simulink model "TST_OilPLmp_DD"  (R2016b)
settings: Solver=FixedStepDiscrete  StartTime=0.0  StopTime=simTime  FixedStep=sampleTime  RelTol=1e-3
values from neighbouring files (symbols this model uses):
  testCase = 1    [initTST_OilPLmp_DD_001.m]    (also in initTST_OilPLmp_DD_002.m = 2)
libraries: simulink x5, UnitTest_Lib x2
settings Model: Creator=xinchangran  LastModifiedBy=xinchangran
settings DebuggingCC: SignalRangeChecking=error

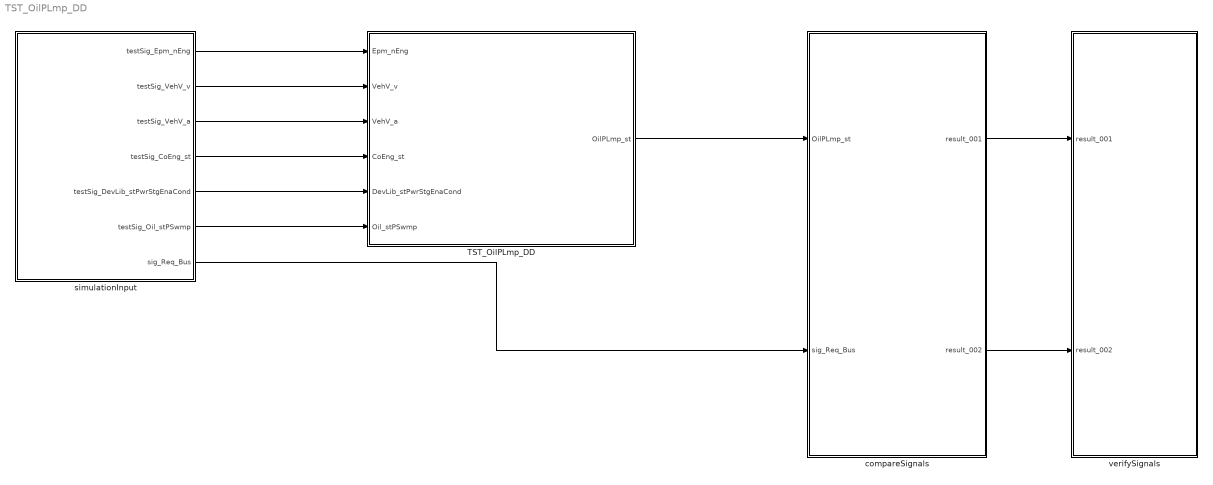
== system TST_OilPLmp_DD ==
  TST_OilPLmp_DD : Subsystem
  compareSignals : Subsystem
  simulationInput : Subsystem
  verifySignals : Subsystem
  wires:
  simulationInput/1(testSig_Epm_nEng) -> TST_OilPLmp_DD/1(Epm_nEng)
  simulationInput/2(testSig_VehV_v) -> TST_OilPLmp_DD/2(VehV_v)
  simulationInput/3(testSig_VehV_a) -> TST_OilPLmp_DD/3(VehV_a)
  simulationInput/4(testSig_CoEng_st) -> TST_OilPLmp_DD/4(CoEng_st)
  simulationInput/5(testSig_DevLib_stPwrStgEnaCond) -> TST_OilPLmp_DD/5(DevLib_stPwrStgEnaCond)
  simulationInput/6(testSig_Oil_stPSwmp) -> TST_OilPLmp_DD/6(Oil_stPSwmp)
  TST_OilPLmp_DD/1(OilPLmp_st) -> compareSignals/1(OilPLmp_st)
  simulationInput/7(sig_Req_Bus) -> compareSignals/2(sig_Req_Bus)
  compareSignals/1(result_001) -> verifySignals/1(result_001)
  compareSignals/2(result_002) -> verifySignals/2(result_002)

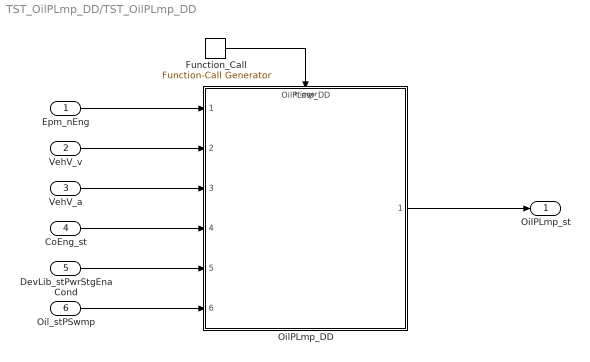
== system TST_OilPLmp_DD/TST_OilPLmp_DD ==
  Epm_nEng : Inport
  VehV_v : Inport  Port=2
  VehV_a : Inport  Port=3
  CoEng_st : Inport  Port=4
  DevLib_stPwrStgEnaCond : Inport  Port=5
  Oil_stPSwmp : Inport  Port=6
  Function_Call : simulink/Ports & Subsystems/Function-Call Generator  sample_time=sampleTime  numberOfIterations=1
  OilPLmp_DD : ModelReference  ModelNameDialog=OilPLmp_DD  SimulationMode=Normal  ModelReferenceVersion=1.211  TriggerPortName=function  TriggerPortTriggerType=function-call  TriggerPortStatesWhenEnabling=held
  OilPLmp_st : Outport
  wires:
  Function_Call/1 -> OilPLmp_DD/Trigger
  Epm_nEng/1 -> OilPLmp_DD/1
  VehV_v/1 -> OilPLmp_DD/2
  VehV_a/1 -> OilPLmp_DD/3
  CoEng_st/1 -> OilPLmp_DD/4
  DevLib_stPwrStgEnaCond/1 -> OilPLmp_DD/5
  Oil_stPSwmp/1 -> OilPLmp_DD/6
  OilPLmp_DD/1 -> OilPLmp_st/1

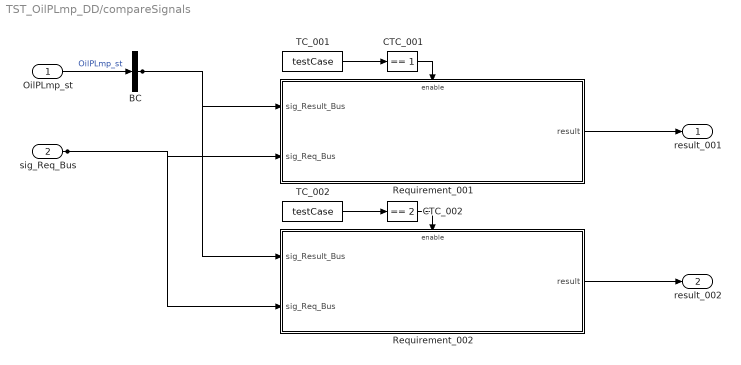
== system TST_OilPLmp_DD/compareSignals ==
  OilPLmp_st : Inport
  sig_Req_Bus : Inport  Port=2
  BC : BusCreator  Inputs=1
  CTC_001 : simulink/Logic and Bit Operations/Compare To Constant  relop===  const=1  OutDataTypeStr=boolean
  CTC_002 : simulink/Logic and Bit Operations/Compare To Constant  relop===  const=2  OutDataTypeStr=boolean
  Requirement_001 : Subsystem
  Requirement_002 : Subsystem
  TC_001 : Constant  Value=testCase
  TC_002 : Constant  Value=testCase
  result_001 : Outport
  result_002 : Outport  Port=2
  wires:
  OilPLmp_st/1 -> BC/1  "OilPLmp_st"
  TC_001/1 -> CTC_001/1
  CTC_001/1 -> Requirement_001/Enable
  sig_Req_Bus/1 -> Requirement_001/2(sig_Req_Bus), Requirement_002/2(sig_Req_Bus)
  BC/1 -> Requirement_001/1(sig_Result_Bus), Requirement_002/1(sig_Result_Bus)
  Requirement_001/1(result) -> result_001/1
  TC_002/1 -> CTC_002/1
  CTC_002/1 -> Requirement_002/Enable
  Requirement_002/1(result) -> result_002/1

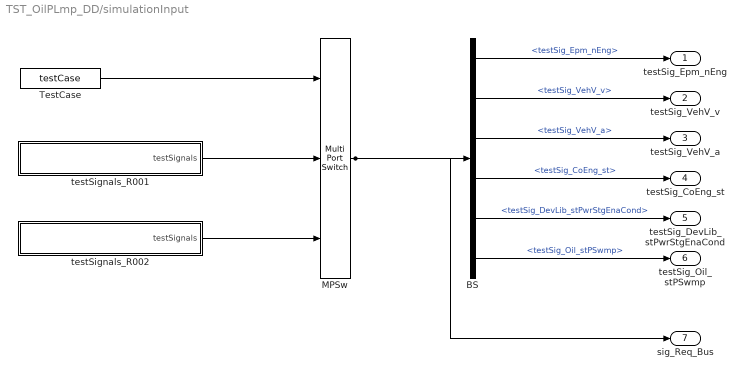
== system TST_OilPLmp_DD/simulationInput ==
  BS : BusSelector  OutputSignals=testSig_Epm_nEng,testSig_VehV_v,testSig_VehV_a,testSig_CoEng_st,testSig_DevLib_stPwrStgEnaCond,testSig_Oil_stPSwmp
  MPSw : MultiPortSwitch  Inputs=2  SaturateOnIntegerOverflow=on  InputSameDT=on
  TestCase : Constant  Value=testCase
  testSignals_R001 : Subsystem
  testSignals_R002 : Subsystem
  testSig_Epm_nEng : Outport
  testSig_VehV_v : Outport  Port=2
  testSig_VehV_a : Outport  Port=3
  testSig_CoEng_st : Outport  Port=4
  testSig_DevLib_stPwrStgEnaCond : Outport  Port=5
  testSig_Oil_stPSwmp : Outport  Port=6
  sig_Req_Bus : Outport  Port=7
  wires:
  BS/1 -> testSig_Epm_nEng/1  "<testSig_Epm_nEng>"
  BS/2 -> testSig_VehV_v/1  "<testSig_VehV_v>"
  BS/3 -> testSig_VehV_a/1  "<testSig_VehV_a>"
  BS/4 -> testSig_CoEng_st/1  "<testSig_CoEng_st>"
  BS/5 -> testSig_DevLib_stPwrStgEnaCond/1  "<testSig_DevLib_stPwrStgEnaCond>"
  BS/6 -> testSig_Oil_stPSwmp/1  "<testSig_Oil_stPSwmp>"
  MPSw/1 -> BS/1, sig_Req_Bus/1
  TestCase/1 -> MPSw/1
  testSignals_R001/1(testSignals) -> MPSw/2
  testSignals_R002/1(testSignals) -> MPSw/3

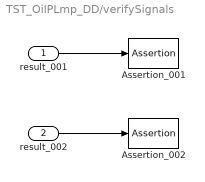
== system TST_OilPLmp_DD/verifySignals ==
  result_001 : Inport
  result_002 : Inport  Port=2
  Assertion_001 : Assertion  Enabled=off
  Assertion_002 : Assertion  Enabled=off
  wires:
  result_001/1 -> Assertion_001/1
  result_002/1 -> Assertion_002/1

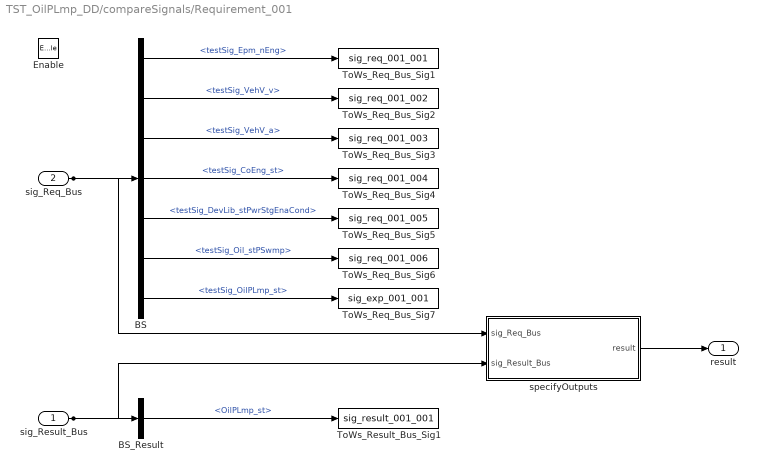
== system TST_OilPLmp_DD/compareSignals/Requirement_001 ==
  sig_Result_Bus : Inport
  sig_Req_Bus : Inport  Port=2
  Enable : EnablePort
  BS : BusSelector  OutputSignals=testSig_Epm_nEng,testSig_VehV_v,testSig_VehV_a,testSig_CoEng_st,testSig_DevLib_stPwrStgEnaCond,testSig_Oil_stPSwmp,testSig_OilPLmp_st
  BS_Result : BusSelector  OutputSignals=OilPLmp_st
  ToWs_Req_Bus_Sig1 : ToWorkspace  VariableName=sig_req_001_001  SaveFormat=Structure With Time
  ToWs_Req_Bus_Sig2 : ToWorkspace  VariableName=sig_req_001_002  SaveFormat=Structure With Time
  ToWs_Req_Bus_Sig3 : ToWorkspace  VariableName=sig_req_001_003  SaveFormat=Structure With Time
  ToWs_Req_Bus_Sig4 : ToWorkspace  VariableName=sig_req_001_004  SaveFormat=Structure With Time
  ToWs_Req_Bus_Sig5 : ToWorkspace  VariableName=sig_req_001_005  SaveFormat=Structure With Time
  ToWs_Req_Bus_Sig6 : ToWorkspace  VariableName=sig_req_001_006  SaveFormat=Structure With Time
  ToWs_Req_Bus_Sig7 : ToWorkspace  VariableName=sig_exp_001_001  SaveFormat=Structure With Time
  ToWs_Result_Bus_Sig1 : ToWorkspace  VariableName=sig_result_001_001  SaveFormat=Structure With Time
  specifyOutputs : Subsystem
  result : Outport
  wires:
  sig_Req_Bus/1 -> BS/1, specifyOutputs/1(sig_Req_Bus)
  BS/1 -> ToWs_Req_Bus_Sig1/1  "<testSig_Epm_nEng>"
  BS/2 -> ToWs_Req_Bus_Sig2/1  "<testSig_VehV_v>"
  BS/3 -> ToWs_Req_Bus_Sig3/1  "<testSig_VehV_a>"
  BS/4 -> ToWs_Req_Bus_Sig4/1  "<testSig_CoEng_st>"
  BS/5 -> ToWs_Req_Bus_Sig5/1  "<testSig_DevLib_stPwrStgEnaCond>"
  BS/6 -> ToWs_Req_Bus_Sig6/1  "<testSig_Oil_stPSwmp>"
  BS/7 -> ToWs_Req_Bus_Sig7/1  "<testSig_OilPLmp_st>"
  sig_Result_Bus/1 -> BS_Result/1, specifyOutputs/2(sig_Result_Bus)
  BS_Result/1 -> ToWs_Result_Bus_Sig1/1  "<OilPLmp_st>"
  specifyOutputs/1(result) -> result/1

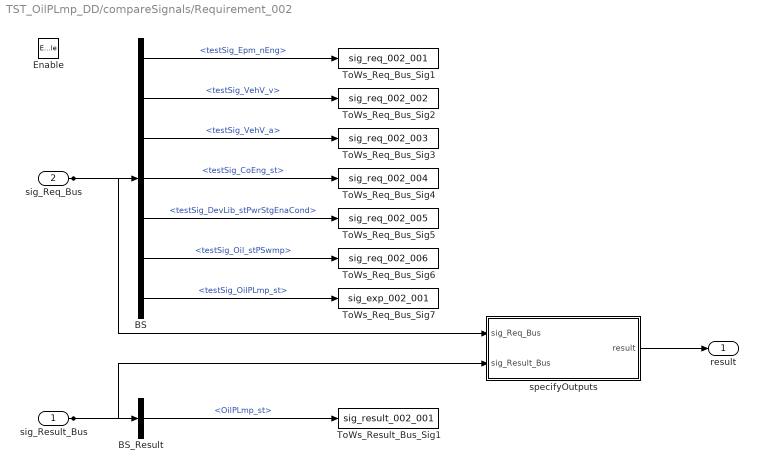
== system TST_OilPLmp_DD/compareSignals/Requirement_002 ==
  sig_Result_Bus : Inport
  sig_Req_Bus : Inport  Port=2
  Enable : EnablePort
  BS : BusSelector  OutputSignals=testSig_Epm_nEng,testSig_VehV_v,testSig_VehV_a,testSig_CoEng_st,testSig_DevLib_stPwrStgEnaCond,testSig_Oil_stPSwmp,testSig_OilPLmp_st
  BS_Result : BusSelector  OutputSignals=OilPLmp_st
  ToWs_Req_Bus_Sig1 : ToWorkspace  VariableName=sig_req_002_001  SaveFormat=Structure With Time
  ToWs_Req_Bus_Sig2 : ToWorkspace  VariableName=sig_req_002_002  SaveFormat=Structure With Time
  ToWs_Req_Bus_Sig3 : ToWorkspace  VariableName=sig_req_002_003  SaveFormat=Structure With Time
  ToWs_Req_Bus_Sig4 : ToWorkspace  VariableName=sig_req_002_004  SaveFormat=Structure With Time
  ToWs_Req_Bus_Sig5 : ToWorkspace  VariableName=sig_req_002_005  SaveFormat=Structure With Time
  ToWs_Req_Bus_Sig6 : ToWorkspace  VariableName=sig_req_002_006  SaveFormat=Structure With Time
  ToWs_Req_Bus_Sig7 : ToWorkspace  VariableName=sig_exp_002_001  SaveFormat=Structure With Time
  ToWs_Result_Bus_Sig1 : ToWorkspace  VariableName=sig_result_002_001  SaveFormat=Structure With Time
  specifyOutputs : Subsystem
  result : Outport
  wires:
  sig_Req_Bus/1 -> BS/1, specifyOutputs/1(sig_Req_Bus)
  BS/1 -> ToWs_Req_Bus_Sig1/1  "<testSig_Epm_nEng>"
  BS/2 -> ToWs_Req_Bus_Sig2/1  "<testSig_VehV_v>"
  BS/3 -> ToWs_Req_Bus_Sig3/1  "<testSig_VehV_a>"
  BS/4 -> ToWs_Req_Bus_Sig4/1  "<testSig_CoEng_st>"
  BS/5 -> ToWs_Req_Bus_Sig5/1  "<testSig_DevLib_stPwrStgEnaCond>"
  BS/6 -> ToWs_Req_Bus_Sig6/1  "<testSig_Oil_stPSwmp>"
  BS/7 -> ToWs_Req_Bus_Sig7/1  "<testSig_OilPLmp_st>"
  sig_Result_Bus/1 -> BS_Result/1, specifyOutputs/2(sig_Result_Bus)
  BS_Result/1 -> ToWs_Result_Bus_Sig1/1  "<OilPLmp_st>"
  specifyOutputs/1(result) -> result/1

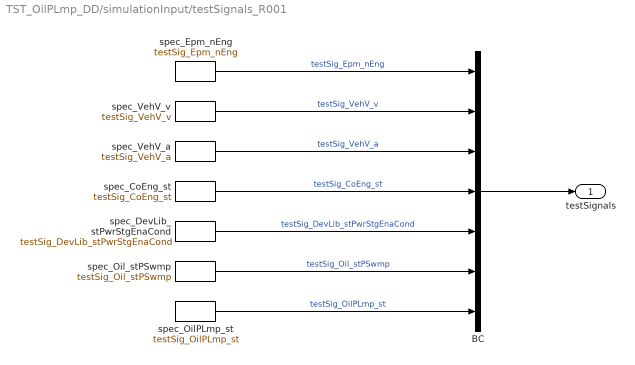
== system TST_OilPLmp_DD/simulationInput/testSignals_R001 ==
  BC : BusCreator  Inputs=7
  spec_CoEng_st : FromWorkspace  VariableName=testSig_CoEng_st  Interpolate=off  OutputAfterFinalValue=Holding final value
  spec_DevLib_stPwrStgEnaCond : FromWorkspace  VariableName=testSig_DevLib_stPwrStgEnaCond  Interpolate=off  OutputAfterFinalValue=Holding final value
  spec_Epm_nEng : FromWorkspace  VariableName=testSig_Epm_nEng  Interpolate=off  OutputAfterFinalValue=Holding final value
  spec_OilPLmp_st : FromWorkspace  VariableName=testSig_OilPLmp_st  Interpolate=off  OutputAfterFinalValue=Holding final value
  spec_Oil_stPSwmp : FromWorkspace  VariableName=testSig_Oil_stPSwmp  Interpolate=off  OutputAfterFinalValue=Holding final value
  spec_VehV_a : FromWorkspace  VariableName=testSig_VehV_a  Interpolate=off  OutputAfterFinalValue=Holding final value
  spec_VehV_v : FromWorkspace  VariableName=testSig_VehV_v  Interpolate=off  OutputAfterFinalValue=Holding final value
  testSignals : Outport
  wires:
  BC/1 -> testSignals/1
  spec_Epm_nEng/1 -> BC/1  "testSig_Epm_nEng"
  spec_VehV_v/1 -> BC/2  "testSig_VehV_v"
  spec_VehV_a/1 -> BC/3  "testSig_VehV_a"
  spec_CoEng_st/1 -> BC/4  "testSig_CoEng_st"
  spec_DevLib_stPwrStgEnaCond/1 -> BC/5  "testSig_DevLib_stPwrStgEnaCond"
  spec_Oil_stPSwmp/1 -> BC/6  "testSig_Oil_stPSwmp"
  spec_OilPLmp_st/1 -> BC/7  "testSig_OilPLmp_st"

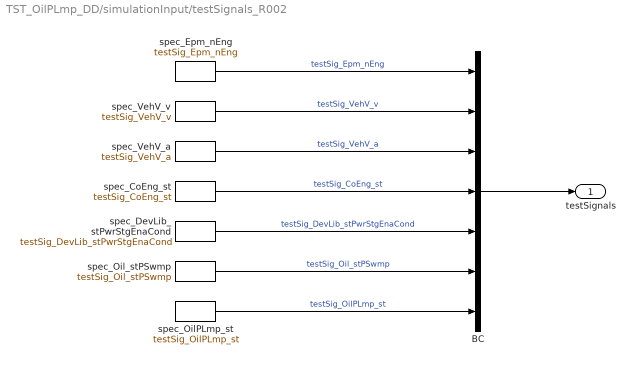
== system TST_OilPLmp_DD/simulationInput/testSignals_R002 ==
  BC : BusCreator  Inputs=7
  spec_CoEng_st : FromWorkspace  VariableName=testSig_CoEng_st  Interpolate=off  OutputAfterFinalValue=Holding final value
  spec_DevLib_stPwrStgEnaCond : FromWorkspace  VariableName=testSig_DevLib_stPwrStgEnaCond  Interpolate=off  OutputAfterFinalValue=Holding final value
  spec_Epm_nEng : FromWorkspace  VariableName=testSig_Epm_nEng  Interpolate=off  OutputAfterFinalValue=Holding final value
  spec_OilPLmp_st : FromWorkspace  VariableName=testSig_OilPLmp_st  Interpolate=off  OutputAfterFinalValue=Holding final value
  spec_Oil_stPSwmp : FromWorkspace  VariableName=testSig_Oil_stPSwmp  Interpolate=off  OutputAfterFinalValue=Holding final value
  spec_VehV_a : FromWorkspace  VariableName=testSig_VehV_a  Interpolate=off  OutputAfterFinalValue=Holding final value
  spec_VehV_v : FromWorkspace  VariableName=testSig_VehV_v  Interpolate=off  OutputAfterFinalValue=Holding final value
  testSignals : Outport
  wires:
  BC/1 -> testSignals/1
  spec_Epm_nEng/1 -> BC/1  "testSig_Epm_nEng"
  spec_VehV_v/1 -> BC/2  "testSig_VehV_v"
  spec_VehV_a/1 -> BC/3  "testSig_VehV_a"
  spec_CoEng_st/1 -> BC/4  "testSig_CoEng_st"
  spec_DevLib_stPwrStgEnaCond/1 -> BC/5  "testSig_DevLib_stPwrStgEnaCond"
  spec_Oil_stPSwmp/1 -> BC/6  "testSig_Oil_stPSwmp"
  spec_OilPLmp_st/1 -> BC/7  "testSig_OilPLmp_st"

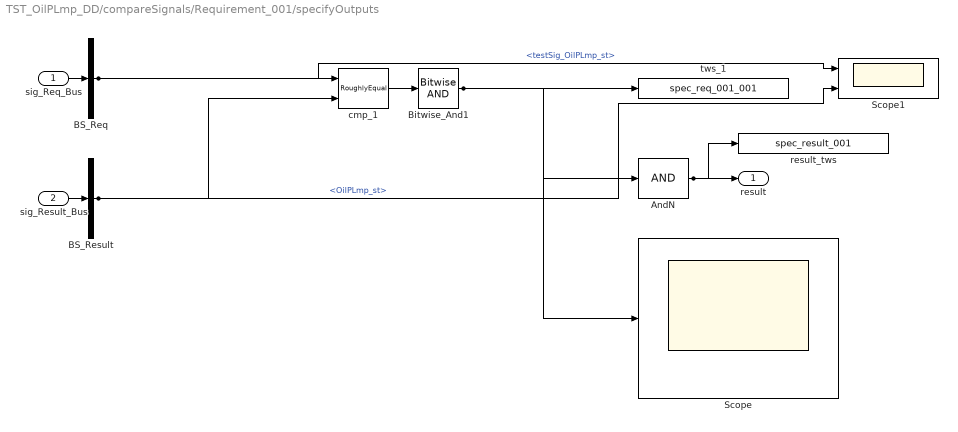
== system TST_OilPLmp_DD/compareSignals/Requirement_001/specifyOutputs ==
  sig_Req_Bus : Inport
  sig_Result_Bus : Inport  Port=2
  AndN : Logic  Inputs=1
  BS_Req : BusSelector  OutputSignals=testSig_OilPLmp_st
  BS_Result : BusSelector  OutputSignals=OilPLmp_st
  Bitwise_And1 : simulink/Logic and Bit Operations/Bitwise Operator  logicop=AND  UseBitMask=off  BitMask=bin2dec('11011001')  BitMaskRealWorld=Stored Integer
  Scope : Scope
  Scope1 : Scope  NumInputPorts=2
  cmp_1 : UnitTest_Lib/RoughlyEqual  slope=0.1
  result_tws : ToWorkspace  VariableName=spec_result_001
  tws_1 : ToWorkspace  VariableName=spec_req_001_001
  result : Outport
  wires:
  sig_Req_Bus/1 -> BS_Req/1
  sig_Result_Bus/1 -> BS_Result/1
  AndN/1 -> result/1, result_tws/1
  BS_Req/1 -> cmp_1/1, Scope1/1  "<testSig_OilPLmp_st>"
  BS_Result/1 -> cmp_1/2, Scope1/2  "<OilPLmp_st>"
  cmp_1/1 -> Bitwise_And1/1
  Bitwise_And1/1 -> tws_1/1, AndN/1, Scope/1

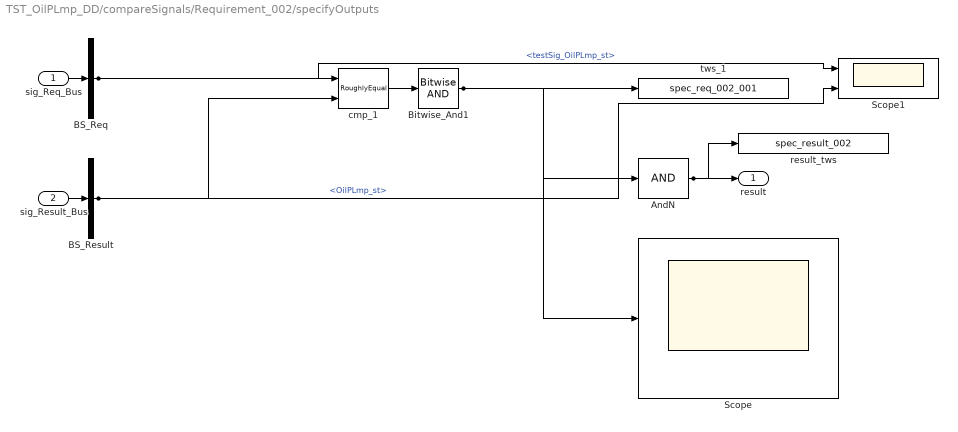
== system TST_OilPLmp_DD/compareSignals/Requirement_002/specifyOutputs ==
  sig_Req_Bus : Inport
  sig_Result_Bus : Inport  Port=2
  AndN : Logic  Inputs=1
  BS_Req : BusSelector  OutputSignals=testSig_OilPLmp_st
  BS_Result : BusSelector  OutputSignals=OilPLmp_st
  Bitwise_And1 : simulink/Logic and Bit Operations/Bitwise Operator  logicop=AND  UseBitMask=off  BitMask=bin2dec('11011001')  BitMaskRealWorld=Stored Integer
  Scope : Scope
  Scope1 : Scope  NumInputPorts=2
  cmp_1 : UnitTest_Lib/RoughlyEqual  slope=0.1
  result_tws : ToWorkspace  VariableName=spec_result_002
  tws_1 : ToWorkspace  VariableName=spec_req_002_001
  result : Outport
  wires:
  sig_Req_Bus/1 -> BS_Req/1
  sig_Result_Bus/1 -> BS_Result/1
  AndN/1 -> result/1, result_tws/1
  BS_Req/1 -> cmp_1/1, Scope1/1  "<testSig_OilPLmp_st>"
  BS_Result/1 -> cmp_1/2, Scope1/2  "<OilPLmp_st>"
  cmp_1/1 -> Bitwise_And1/1
  Bitwise_And1/1 -> tws_1/1, AndN/1, Scope/1
